simulink model "stormAD_Architecture_v1"  (R2024a)
settings: Solver=FixedStepDiscrete  StartTime=0.0  StopTime=10.0  RelTol=1e-3
model workspace (MAT data in the model file):
  bstInterface : Simulink.Bus (value not decoded)
undefined symbols (not defined in the file): orig, RepoFilePath, UI, VisualizeDataset
(part 2 of 3)

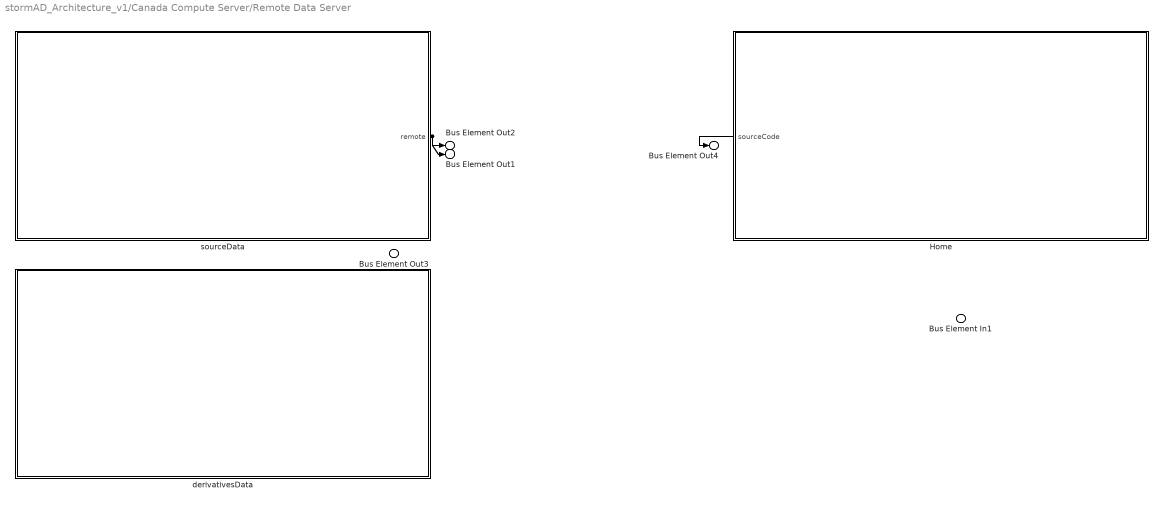
== system stormAD_Architecture_v1/Canada Compute Server/Remote Data Server ==
  Bus Element In1 : Inport  PortName=Derivatives
  " sourceData" : Subsystem
      settings: PortSchema="{\"entries\":[{\"content\":{\"headerSize\":26,\"margin\":15,\"minimumSpacing\":25,\"sides\":[{\"content\":{},\"type\":\"ConnectorPlacement.EquallySpacedRectSide\",\"uuid\":\"a3539b9a-22db-4da3-b271-35b287ced3a1\"},{\"content\":{\"connectorIds\":[\"Out1\"],\"side\":\"RIGHT\"},\"type\":\"ConnectorPlacement.EquallySpacedRectSide\",\"uuid\":\"72d9f298-5062-46d4-b3c5-f2fa85d7a7a6\"},{\"content\":{\"side\":\"TOP\"},\"type\":\"ConnectorPlacement.EquallySpacedRectSide\",\"uuid\":\"050469fd-3881-4b53-a813-94df038aa659\"}]},\"type\":\"ConnectorPlacement.EquallySpacedConnector\",\"uuid\":\"6db04dad-62f3-4987-a6a9-d236db4fe2a3\"}],\"packageUris\":[\"http://schema.mathworks.com/mf0/Connector/R2020b\"],\"version\":\"1.0\"}"
  Home : Subsystem
      settings: PortSchema="{\"entries\":[{\"content\":{\"headerSize\":26,\"margin\":15,\"minimumSpacing\":25,\"sides\":[{\"content\":{\"connectorIds\":[\"Out1\"]},\"type\":\"ConnectorPlacement.EquallySpacedRectSide\",\"uuid\":\"a3539b9a-22db-4da3-b271-35b287ced3a1\"},{\"content\":{\"side\":\"RIGHT\"},\"type\":\"ConnectorPlacement.EquallySpacedRectSide\",\"uuid\":\"72d9f298-5062-46d4-b3c5-f2fa85d7a7a6\"},{\"content\":{\"side\":\"TOP\"},\"type\":\"ConnectorPlacement.EquallySpacedRectSide\",\"uuid\":\"050469fd-3881-4b53-a813-94df038aa659\"}]},\"type\":\"ConnectorPlacement.EquallySpacedConnector\",\"uuid\":\"6db04dad-62f3-4987-a6a9-d236db4fe2a3\"}],\"packageUris\":[\"http://schema.mathworks.com/mf0/Connector/R2020b\"],\"version\":\"1.0\"}"
  derivativesData : Subsystem
      settings: PortSchema="{\"entries\":[{\"content\":{\"headerSize\":26,\"margin\":15,\"minimumSpacing\":25,\"sides\":[{\"content\":{},\"type\":\"ConnectorPlacement.EquallySpacedRectSide\",\"uuid\":\"a3539b9a-22db-4da3-b271-35b287ced3a1\"},{\"content\":{\"side\":\"RIGHT\"},\"type\":\"ConnectorPlacement.EquallySpacedRectSide\",\"uuid\":\"72d9f298-5062-46d4-b3c5-f2fa85d7a7a6\"},{\"content\":{\"side\":\"TOP\"},\"type\":\"ConnectorPlacement.EquallySpacedRectSide\",\"uuid\":\"050469fd-3881-4b53-a813-94df038aa659\"}]},\"type\":\"ConnectorPlacement.EquallySpacedConnector\",\"uuid\":\"6db04dad-62f3-4987-a6a9-d236db4fe2a3\"}],\"packageUris\":[\"http://schema.mathworks.com/mf0/Connector/R2020b\"],\"version\":\"1.0\"}"
  Bus Element Out4 : Outport  AllowServiceAccess=on  PortName=sourceCode  Element=github
  Bus Element Out3 : Outport  Port=2  AllowServiceAccess=on  PortName=SSHPort
  Bus Element Out1 : Outport  Port=3  AllowServiceAccess=on  PortName=remote.raw
  Bus Element Out2 : Outport  Port=4  AllowServiceAccess=on  PortName=remote.derivatives
  wires:
  " sourceData"/1(remote) -> Bus Element Out1/1, Bus Element Out2/1
  Home/1(sourceCode) -> Bus Element Out4/1

== system stormAD_Architecture_v1/Canada Compute Server/create Virtual Environment ==

== system stormAD_Architecture_v1/Canada Compute Server/gitClone Brainstorm ==
  Bus Element In1 : Inport  AllowServiceAccess=on  PortName=sourceCode

== system stormAD_Architecture_v1/Canada Compute Server/jobScheduler ==

== system stormAD_Architecture_v1/Canada Compute Server/loadPython ==

== system stormAD_Architecture_v1/Canada Compute Server/processingSoftware ==

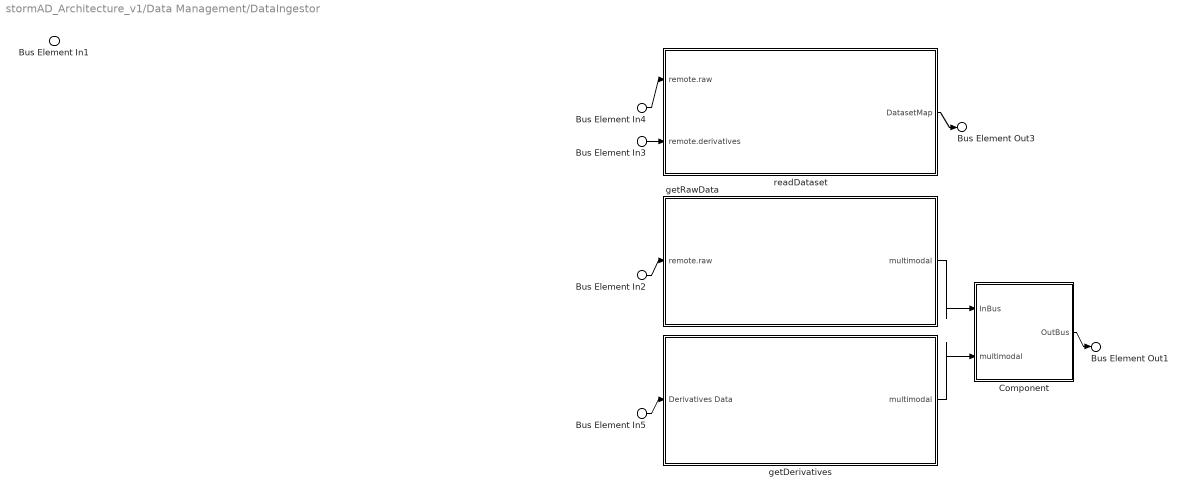
== system stormAD_Architecture_v1/Data Management/DataIngestor ==
  Bus Element In2 : Inport  AllowServiceAccess=on  PortName=remote.raw
  Bus Element In4 : Inport  AllowServiceAccess=on  PortName=remote.raw
  Bus Element In3 : Inport  Port=2  AllowServiceAccess=on  PortName=remote.derivatives
  Bus Element In5 : Inport  Port=2  AllowServiceAccess=on  PortName=remote.derivatives
  Bus Element In1 : Inport  Port=3  PortName=DataRequest
  Component : Subsystem
      settings: PortSchema="{\"entries\":[{\"content\":{\"headerSize\":26,\"margin\":15,\"minimumSpacing\":25,\"sides\":[{\"content\":{\"connectorIds\":[\"In1\",\"In2\"]},\"type\":\"ConnectorPlacement.EquallySpacedRectSide\",\"uuid\":\"a3539b9a-22db-4da3-b271-35b287ced3a1\"},{\"content\":{\"connectorIds\":[\"Out1\"],\"side\":\"RIGHT\"},\"type\":\"ConnectorPlacement.EquallySpacedRectSide\",\"uuid\":\"72d9f298-5062-46d4-b3c5-f2fa85d7a7a6\"},{\"content\":{\"side\":\"TOP\"},\"type\":\"ConnectorPlacement.EquallySpacedRectSide\",\"uuid\":\"050469fd-3881-4b53-a813-94df038aa659\"}]},\"type\":\"ConnectorPlacement.EquallySpacedConnector\",\"uuid\":\"6db04dad-62f3-4987-a6a9-d236db4fe2a3\"}],\"packageUris\":[\"http://schema.mathworks.com/mf0/Connector/R2020b\"],\"version\":\"1.0\"}"
  getDerivatives : Subsystem
      settings: PortSchema="{\"entries\":[{\"content\":{\"headerSize\":26,\"margin\":15,\"minimumSpacing\":25,\"sides\":[{\"content\":{\"connectorIds\":[\"In1\"]},\"type\":\"ConnectorPlacement.EquallySpacedRectSide\",\"uuid\":\"d99db108-8c8a-4010-81b2-f142fbf318f5\"},{\"content\":{\"connectorIds\":[\"Out1\"],\"side\":\"RIGHT\"},\"type\":\"ConnectorPlacement.EquallySpacedRectSide\",\"uuid\":\"9190d96c-22e3-4cc9-a507-8f094dc67743\"},{\"content\":{\"side\":\"TOP\"},\"type\":\"ConnectorPlacement.EquallySpacedRectSide\",\"uuid\":\"08b46875-eac1-4edb-b2eb-5598dd517a75\"}]},\"type\":\"ConnectorPlacement.EquallySpacedConnector\",\"uuid\":\"c8d2d02b-cf5a-431f-8876-22d36c8a9b33\"}],\"packageUris\":[\"http://schema.mathworks.com/mf0/Connector/R2020b\"],\"version\":\"1.0\"}"
  getRawData : Subsystem
      settings: PortSchema="{\"entries\":[{\"content\":{\"headerSize\":26,\"margin\":15,\"minimumSpacing\":25,\"sides\":[{\"content\":{\"connectorIds\":[\"In1\"]},\"type\":\"ConnectorPlacement.EquallySpacedRectSide\",\"uuid\":\"d99db108-8c8a-4010-81b2-f142fbf318f5\"},{\"content\":{\"connectorIds\":[\"Out1\"],\"side\":\"RIGHT\"},\"type\":\"ConnectorPlacement.EquallySpacedRectSide\",\"uuid\":\"9190d96c-22e3-4cc9-a507-8f094dc67743\"},{\"content\":{\"side\":\"TOP\"},\"type\":\"ConnectorPlacement.EquallySpacedRectSide\",\"uuid\":\"08b46875-eac1-4edb-b2eb-5598dd517a75\"}]},\"type\":\"ConnectorPlacement.EquallySpacedConnector\",\"uuid\":\"c8d2d02b-cf5a-431f-8876-22d36c8a9b33\"}],\"packageUris\":[\"http://schema.mathworks.com/mf0/Connector/R2020b\"],\"version\":\"1.0\"}"
  readDataset : Subsystem
      settings: PortSchema="{\"entries\":[{\"content\":{\"headerSize\":26,\"margin\":15,\"minimumSpacing\":25,\"sides\":[{\"content\":{\"connectorIds\":[\"In1\",\"In2\"]},\"type\":\"ConnectorPlacement.EquallySpacedRectSide\",\"uuid\":\"d99db108-8c8a-4010-81b2-f142fbf318f5\"},{\"content\":{\"connectorIds\":[\"Out1\"],\"side\":\"RIGHT\"},\"type\":\"ConnectorPlacement.EquallySpacedRectSide\",\"uuid\":\"9190d96c-22e3-4cc9-a507-8f094dc67743\"},{\"content\":{\"side\":\"TOP\"},\"type\":\"ConnectorPlacement.EquallySpacedRectSide\",\"uuid\":\"08b46875-eac1-4edb-b2eb-5598dd517a75\"}]},\"type\":\"ConnectorPlacement.EquallySpacedConnector\",\"uuid\":\"c8d2d02b-cf5a-431f-8876-22d36c8a9b33\"}],\"packageUris\":[\"http://schema.mathworks.com/mf0/Connector/R2020b\"],\"version\":\"1.0\"}"
  Bus Element Out1 : Outport  PortName=remote
  Bus Element Out3 : Outport  Port=2  PortName=DatasetMap
  wires:
  readDataset/1(DatasetMap) -> Bus Element Out3/1
  Bus Element In2/1 -> getRawData/1(remote.raw)
  Bus Element In4/1 -> readDataset/1(remote.raw)
  Bus Element In3/1 -> readDataset/2(remote.derivatives)
  Bus Element In5/1 -> getDerivatives/1(Derivatives Data)
  getDerivatives/1(multimodal) -> Component/2(multimodal)
  getRawData/1(multimodal) -> Component/1(InBus)
  Component/1(OutBus) -> Bus Element Out1/1

== system stormAD_Architecture_v1/Data Management/Database Server ==
  Bus Element In2 : Inport  PortName=DerivativesMetadata
  Bus Element In3 : Inport  Port=2  PortName=Local Derivatives Metadata
  Bus Element In1 : Inport  Port=3  PortName=Dataset Metadata
  Bus Element Out1 : Outport  AllowServiceAccess=on  PortName=Metadata

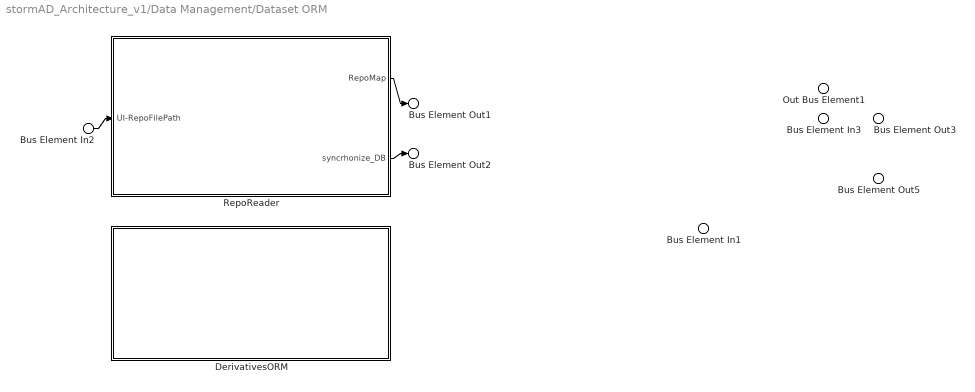
== system stormAD_Architecture_v1/Data Management/Dataset ORM ==
  Bus Element In3 : Inport  PortName=DatasetMap
  Bus Element In2 : Inport  Port=2  PortName=UI-RepoFilePath
  Bus Element In1 : Inport  Port=3  AllowServiceAccess=on  PortName=Metadata
  DerivativesORM : Subsystem
      settings: PortSchema="{\"entries\":[{\"content\":{\"headerSize\":26,\"margin\":15,\"minimumSpacing\":25,\"sides\":[{\"content\":{},\"type\":\"ConnectorPlacement.EquallySpacedRectSide\",\"uuid\":\"d99db108-8c8a-4010-81b2-f142fbf318f5\"},{\"content\":{\"side\":\"RIGHT\"},\"type\":\"ConnectorPlacement.EquallySpacedRectSide\",\"uuid\":\"9190d96c-22e3-4cc9-a507-8f094dc67743\"},{\"content\":{\"side\":\"TOP\"},\"type\":\"ConnectorPlacement.EquallySpacedRectSide\",\"uuid\":\"08b46875-eac1-4edb-b2eb-5598dd517a75\"}]},\"type\":\"ConnectorPlacement.EquallySpacedConnector\",\"uuid\":\"c8d2d02b-cf5a-431f-8876-22d36c8a9b33\"}],\"packageUris\":[\"http://schema.mathworks.com/mf0/Connector/R2020b\"],\"version\":\"1.0\"}"
  RepoReader : Subsystem
      settings: PortSchema="{\"entries\":[{\"content\":{\"headerSize\":26,\"margin\":15,\"minimumSpacing\":25,\"sides\":[{\"content\":{\"connectorIds\":[\"In1\"]},\"type\":\"ConnectorPlacement.EquallySpacedRectSide\",\"uuid\":\"d99db108-8c8a-4010-81b2-f142fbf318f5\"},{\"content\":{\"connectorIds\":[\"Out1\",\"Out2\"],\"side\":\"RIGHT\"},\"type\":\"ConnectorPlacement.EquallySpacedRectSide\",\"uuid\":\"9190d96c-22e3-4cc9-a507-8f094dc67743\"},{\"content\":{\"side\":\"TOP\"},\"type\":\"ConnectorPlacement.EquallySpacedRectSide\",\"uuid\":\"08b46875-eac1-4edb-b2eb-5598dd517a75\"}]},\"type\":\"ConnectorPlacement.EquallySpacedConnector\",\"uuid\":\"c8d2d02b-cf5a-431f-8876-22d36c8a9b33\"}],\"packageUris\":[\"http://schema.mathworks.com/mf0/Connector/R2020b\"],\"version\":\"1.0\"}"
  Bus Element Out5 : Outport  PortName=DerivativesMetadata
  Bus Element Out2 : Outport  Port=2  PortName=syncrhonize_DB
  Bus Element Out3 : Outport  Port=3  PortName=DataRequest
  Bus Element Out1 : Outport  Port=4  PortName=RepoMap
  Out Bus Element1 : Outport  Port=5  PortName=UI-VisualizeDataset
  wires:
  Bus Element In2/1 -> RepoReader/1(UI-RepoFilePath)
  RepoReader/1(RepoMap) -> Bus Element Out1/1
  RepoReader/2(syncrhonize_DB) -> Bus Element Out2/1

== system stormAD_Architecture_v1/Local Data Server/UserDir ==
  Bus Element Out1 : Outport  AllowServiceAccess=on  PortName=userConfigRemote

== system stormAD_Architecture_v1/Local Data Server/brainstorm3 ==

== system stormAD_Architecture_v1/Local Data Server/brainstorm_db ==
  Bus Element In1 : Inport  AllowServiceAccess=on  PortName=Derivatives

== system stormAD_Architecture_v1/Local Data Server/remoteConfig ==
  Bus Element Out1 : Outport  AllowServiceAccess=on  PortName=userConfigRemote

== system stormAD_Architecture_v1/Local Data Server/sourceData ==
  Bus Element In2 : Inport  AllowServiceAccess=on  PortName=StormDerivatives
  Bus Element In1 : Inport  Port=2  PortName=remote
  Out Bus Element1 : Outport  PortName=local

== system stormAD_Architecture_v1/Remote Data Connect/LORIS Data Ingestor ==

== system stormAD_Architecture_v1/Remote Data Connect/Linux ==
  Bus Element In1 : Inport  AllowServiceAccess=on  PortName=Client

== system stormAD_Architecture_v1/Remote Data Connect/Windows ==
  Bus Element In1 : Inport  AllowServiceAccess=on  PortName=Client

== system stormAD_Architecture_v1/Remote Data Connect/gitClone Brainstorm ==
  Bus Element In1 : Inport  AllowServiceAccess=on  PortName=sourceCode

== system stormAD_Architecture_v1/StormAD Core/Anatomy ==
  Bus Element In1 : Inport  PortName=anat
  Bus Element Out1 : Outport  PortName=anat4pet
  Bus Element Out2 : Outport  Port=2  PortName=anat4meg
  Bus Element Out3 : Outport  Port=3  PortName=anatMetadata
  Bus Element Out4 : Outport  Port=4  PortName=anatDerivs

== system stormAD_Architecture_v1/StormAD Core/MEG ==
  Bus Element In2 : Inport  PortName=anat4meg
  Bus Element In1 : Inport  Port=2  PortName=meg
  featureExtractionModule : Subsystem
      settings: PortSchema="{\"entries\":[{\"content\":{\"headerSize\":26,\"margin\":15,\"minimumSpacing\":25,\"sides\":[{\"content\":{},\"type\":\"ConnectorPlacement.EquallySpacedRectSide\",\"uuid\":\"a3539b9a-22db-4da3-b271-35b287ced3a1\"},{\"content\":{\"side\":\"RIGHT\"},\"type\":\"ConnectorPlacement.EquallySpacedRectSide\",\"uuid\":\"72d9f298-5062-46d4-b3c5-f2fa85d7a7a6\"},{\"content\":{\"side\":\"TOP\"},\"type\":\"ConnectorPlacement.EquallySpacedRectSide\",\"uuid\":\"050469fd-3881-4b53-a813-94df038aa659\"}]},\"type\":\"ConnectorPlacement.EquallySpacedConnector\",\"uuid\":\"6db04dad-62f3-4987-a6a9-d236db4fe2a3\"}],\"packageUris\":[\"http://schema.mathworks.com/mf0/Connector/R2020b\"],\"version\":\"1.0\"}"
  Bus Element Out1 : Outport  PortName=megMetadata
  Bus Element Out2 : Outport  Port=2  PortName=megSurf
  Bus Element Out3 : Outport  Port=3  PortName=megDerivs

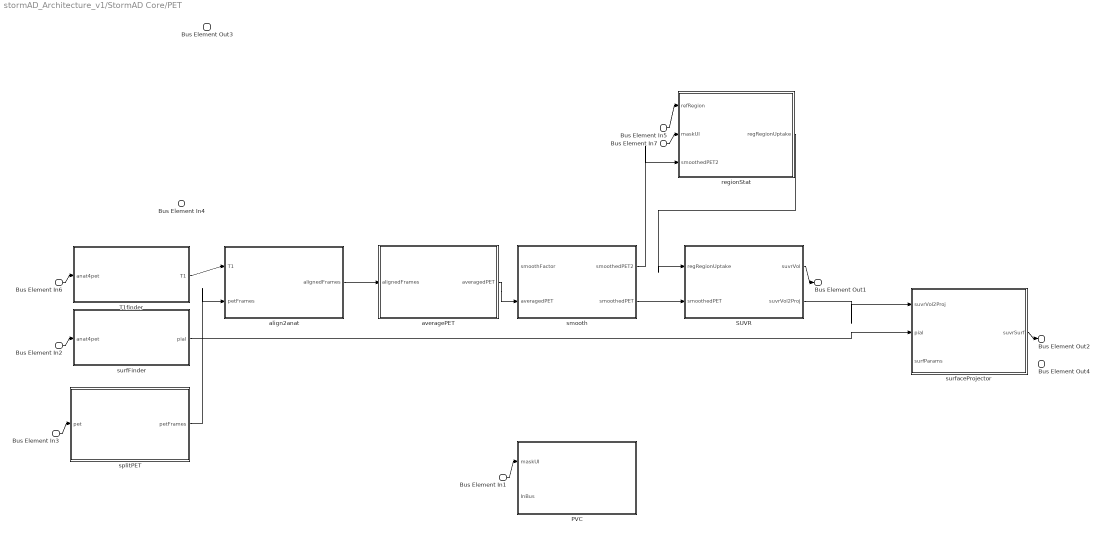
== system stormAD_Architecture_v1/StormAD Core/PET ==
  Bus Element In7 : Inport  PortName=maskUI
  Bus Element In1 : Inport  PortName=maskUI
  Bus Element In5 : Inport  Port=2  PortName=anat4pet
  Bus Element In6 : Inport  Port=2  PortName=anat4pet
  Bus Element In2 : Inport  Port=2  PortName=anat4pet
  Bus Element In4 : Inport  Port=2  PortName=anat4pet  Element=signal1
  Bus Element In3 : Inport  Port=3  PortName=pet
  PVC : Subsystem
      settings: PortSchema="{\"entries\":[{\"content\":{\"headerSize\":26,\"margin\":15,\"minimumSpacing\":25,\"sides\":[{\"content\":{\"connectorIds\":[\"In1\",\"In2\"]},\"type\":\"ConnectorPlacement.EquallySpacedRectSide\",\"uuid\":\"a3539b9a-22db-4da3-b271-35b287ced3a1\"},{\"content\":{\"side\":\"RIGHT\"},\"type\":\"ConnectorPlacement.EquallySpacedRectSide\",\"uuid\":\"72d9f298-5062-46d4-b3c5-f2fa85d7a7a6\"},{\"content\":{\"side\":\"TOP\"},\"type\":\"ConnectorPlacement.EquallySpacedRectSide\",\"uuid\":\"050469fd-3881-4b53-a813-94df038aa659\"}]},\"type\":\"ConnectorPlacement.EquallySpacedConnector\",\"uuid\":\"6db04dad-62f3-4987-a6a9-d236db4fe2a3\"}],\"packageUris\":[\"http://schema.mathworks.com/mf0/Connector/R2020b\"],\"version\":\"1.0\"}"
  SUVR : Subsystem
      settings: PortSchema="{\"entries\":[{\"content\":{\"headerSize\":26,\"margin\":15,\"minimumSpacing\":25,\"sides\":[{\"content\":{\"connectorIds\":[\"In1\",\"In2\"]},\"type\":\"ConnectorPlacement.EquallySpacedRectSide\",\"uuid\":\"a3539b9a-22db-4da3-b271-35b287ced3a1\"},{\"content\":{\"connectorIds\":[\"Out1\",\"Out2\"],\"side\":\"RIGHT\"},\"type\":\"ConnectorPlacement.EquallySpacedRectSide\",\"uuid\":\"72d9f298-5062-46d4-b3c5-f2fa85d7a7a6\"},{\"content\":{\"side\":\"TOP\"},\"type\":\"ConnectorPlacement.EquallySpacedRectSide\",\"uuid\":\"050469fd-3881-4b53-a813-94df038aa659\"}]},\"type\":\"ConnectorPlacement.EquallySpacedConnector\",\"uuid\":\"6db04dad-62f3-4987-a6a9-d236db4fe2a3\"}],\"packageUris\":[\"http://schema.mathworks.com/mf0/Connector/R2020b\"],\"version\":\"1.0\"}"
  T1finder : Subsystem
      settings: PortSchema="{\"entries\":[{\"content\":{\"headerSize\":26,\"margin\":15,\"minimumSpacing\":25,\"sides\":[{\"content\":{\"connectorIds\":[\"In1\"]},\"type\":\"ConnectorPlacement.EquallySpacedRectSide\",\"uuid\":\"a3539b9a-22db-4da3-b271-35b287ced3a1\"},{\"content\":{\"connectorIds\":[\"Out1\"],\"side\":\"RIGHT\"},\"type\":\"ConnectorPlacement.EquallySpacedRectSide\",\"uuid\":\"72d9f298-5062-46d4-b3c5-f2fa85d7a7a6\"},{\"content\":{\"side\":\"TOP\"},\"type\":\"ConnectorPlacement.EquallySpacedRectSide\",\"uuid\":\"050469fd-3881-4b53-a813-94df038aa659\"},{\"content\":{\"side\":\"BOTTOM\"},\"type\":\"ConnectorPlacement.EquallySpacedRectSide\",\"uuid\":\"a1469e70-16e5-4ce1-b6fd-4b50fed9e5f8\"}]},\"type\":\"ConnectorPlacement.EquallySpacedConnector\",\"uuid\":\"6db04dad-62f3-4987-a6a9-d236db4fe2a3\"}],\"packageUris\":[\"http://schema.mathworks.com/mf0/Connector/R2020b\"],\"version\":\"1.0\"}"
  align2anat : Subsystem
      settings: PortSchema="{\"entries\":[{\"content\":{\"headerSize\":26,\"margin\":15,\"minimumSpacing\":25,\"sides\":[{\"content\":{\"connectorIds\":[\"In1\",\"In2\"]},\"type\":\"ConnectorPlacement.EquallySpacedRectSide\",\"uuid\":\"a3539b9a-22db-4da3-b271-35b287ced3a1\"},{\"content\":{\"connectorIds\":[\"Out1\"],\"side\":\"RIGHT\"},\"type\":\"ConnectorPlacement.EquallySpacedRectSide\",\"uuid\":\"72d9f298-5062-46d4-b3c5-f2fa85d7a7a6\"},{\"content\":{\"side\":\"TOP\"},\"type\":\"ConnectorPlacement.EquallySpacedRectSide\",\"uuid\":\"050469fd-3881-4b53-a813-94df038aa659\"}]},\"type\":\"ConnectorPlacement.EquallySpacedConnector\",\"uuid\":\"6db04dad-62f3-4987-a6a9-d236db4fe2a3\"}],\"packageUris\":[\"http://schema.mathworks.com/mf0/Connector/R2020b\"],\"version\":\"1.0\"}"
  averagePET : Subsystem
      settings: PortSchema="{\"entries\":[{\"content\":{\"headerSize\":26,\"margin\":15,\"minimumSpacing\":25,\"sides\":[{\"content\":{\"connectorIds\":[\"In1\"]},\"type\":\"ConnectorPlacement.EquallySpacedRectSide\",\"uuid\":\"a3539b9a-22db-4da3-b271-35b287ced3a1\"},{\"content\":{\"connectorIds\":[\"Out1\"],\"side\":\"RIGHT\"},\"type\":\"ConnectorPlacement.EquallySpacedRectSide\",\"uuid\":\"72d9f298-5062-46d4-b3c5-f2fa85d7a7a6\"},{\"content\":{\"side\":\"TOP\"},\"type\":\"ConnectorPlacement.EquallySpacedRectSide\",\"uuid\":\"050469fd-3881-4b53-a813-94df038aa659\"}]},\"type\":\"ConnectorPlacement.EquallySpacedConnector\",\"uuid\":\"6db04dad-62f3-4987-a6a9-d236db4fe2a3\"}],\"packageUris\":[\"http://schema.mathworks.com/mf0/Connector/R2020b\"],\"version\":\"1.0\"}"
  regionStat : Subsystem
      settings: PortSchema="{\"entries\":[{\"content\":{\"headerSize\":26,\"margin\":15,\"minimumSpacing\":25,\"sides\":[{\"content\":{\"connectorIds\":[\"In1\",\"In2\",\"In3\"]},\"type\":\"ConnectorPlacement.EquallySpacedRectSide\",\"uuid\":\"a3539b9a-22db-4da3-b271-35b287ced3a1\"},{\"content\":{\"connectorIds\":[\"Out1\"],\"side\":\"RIGHT\"},\"type\":\"ConnectorPlacement.EquallySpacedRectSide\",\"uuid\":\"72d9f298-5062-46d4-b3c5-f2fa85d7a7a6\"},{\"content\":{\"side\":\"TOP\"},\"type\":\"ConnectorPlacement.EquallySpacedRectSide\",\"uuid\":\"050469fd-3881-4b53-a813-94df038aa659\"}]},\"type\":\"ConnectorPlacement.EquallySpacedConnector\",\"uuid\":\"6db04dad-62f3-4987-a6a9-d236db4fe2a3\"}],\"packageUris\":[\"http://schema.mathworks.com/mf0/Connector/R2020b\"],\"version\":\"1.0\"}"
  smooth : Subsystem
      settings: PortSchema="{\"entries\":[{\"content\":{\"headerSize\":26,\"margin\":15,\"minimumSpacing\":25,\"sides\":[{\"content\":{\"connectorIds\":[\"In1\",\"In2\"]},\"type\":\"ConnectorPlacement.EquallySpacedRectSide\",\"uuid\":\"a3539b9a-22db-4da3-b271-35b287ced3a1\"},{\"content\":{\"connectorIds\":[\"Out1\",\"Out2\"],\"side\":\"RIGHT\"},\"type\":\"ConnectorPlacement.EquallySpacedRectSide\",\"uuid\":\"72d9f298-5062-46d4-b3c5-f2fa85d7a7a6\"},{\"content\":{\"side\":\"TOP\"},\"type\":\"ConnectorPlacement.EquallySpacedRectSide\",\"uuid\":\"050469fd-3881-4b53-a813-94df038aa659\"}]},\"type\":\"ConnectorPlacement.EquallySpacedConnector\",\"uuid\":\"6db04dad-62f3-4987-a6a9-d236db4fe2a3\"}],\"packageUris\":[\"http://schema.mathworks.com/mf0/Connector/R2020b\"],\"version\":\"1.0\"}"
  splitPET : Subsystem
      settings: PortSchema="{\"entries\":[{\"content\":{\"headerSize\":26,\"margin\":15,\"minimumSpacing\":25,\"sides\":[{\"content\":{\"connectorIds\":[\"In1\"]},\"type\":\"ConnectorPlacement.EquallySpacedRectSide\",\"uuid\":\"a3539b9a-22db-4da3-b271-35b287ced3a1\"},{\"content\":{\"connectorIds\":[\"Out1\"],\"side\":\"RIGHT\"},\"type\":\"ConnectorPlacement.EquallySpacedRectSide\",\"uuid\":\"72d9f298-5062-46d4-b3c5-f2fa85d7a7a6\"},{\"content\":{\"side\":\"TOP\"},\"type\":\"ConnectorPlacement.EquallySpacedRectSide\",\"uuid\":\"050469fd-3881-4b53-a813-94df038aa659\"}]},\"type\":\"ConnectorPlacement.EquallySpacedConnector\",\"uuid\":\"6db04dad-62f3-4987-a6a9-d236db4fe2a3\"}],\"packageUris\":[\"http://schema.mathworks.com/mf0/Connector/R2020b\"],\"version\":\"1.0\"}"
  surfFinder : Subsystem
      settings: PortSchema="{\"entries\":[{\"content\":{\"headerSize\":26,\"margin\":15,\"minimumSpacing\":25,\"sides\":[{\"content\":{\"connectorIds\":[\"In1\"]},\"type\":\"ConnectorPlacement.EquallySpacedRectSide\",\"uuid\":\"a3539b9a-22db-4da3-b271-35b287ced3a1\"},{\"content\":{\"connectorIds\":[\"Out1\"],\"side\":\"RIGHT\"},\"type\":\"ConnectorPlacement.EquallySpacedRectSide\",\"uuid\":\"72d9f298-5062-46d4-b3c5-f2fa85d7a7a6\"},{\"content\":{\"side\":\"TOP\"},\"type\":\"ConnectorPlacement.EquallySpacedRectSide\",\"uuid\":\"050469fd-3881-4b53-a813-94df038aa659\"}]},\"type\":\"ConnectorPlacement.EquallySpacedConnector\",\"uuid\":\"6db04dad-62f3-4987-a6a9-d236db4fe2a3\"}],\"packageUris\":[\"http://schema.mathworks.com/mf0/Connector/R2020b\"],\"version\":\"1.0\"}"
  surfaceProjector : Subsystem
      settings: PortSchema="{\"entries\":[{\"content\":{\"headerSize\":26,\"margin\":15,\"minimumSpacing\":25,\"sides\":[{\"content\":{\"connectorIds\":[\"In1\",\"In3\",\"In2\"]},\"type\":\"ConnectorPlacement.EquallySpacedRectSide\",\"uuid\":\"a3539b9a-22db-4da3-b271-35b287ced3a1\"},{\"content\":{\"connectorIds\":[\"Out1\"],\"side\":\"RIGHT\"},\"type\":\"ConnectorPlacement.EquallySpacedRectSide\",\"uuid\":\"72d9f298-5062-46d4-b3c5-f2fa85d7a7a6\"},{\"content\":{\"side\":\"TOP\"},\"type\":\"ConnectorPlacement.EquallySpacedRectSide\",\"uuid\":\"050469fd-3881-4b53-a813-94df038aa659\"},{\"content\":{\"side\":\"BOTTOM\"},\"type\":\"ConnectorPlacement.EquallySpacedRectSide\",\"uuid\":\"ca80c562-ab11-42f8-9713-788a61e6aac3\"}]},\"type\":\"ConnectorPlacement.EquallySpacedConnector\",\"uuid\":\"6db04dad-62f3-4987-a6a9-d236db4fe2a3\"}],\"packageUris\":[\"http://schema.mathworks.com/mf0/Connector/R2020b\"],\"version\":\"1.0\"}"
  Bus Element Out3 : Outport  PortName=petMedata
  Bus Element Out1 : Outport  Port=2  PortName=suvrVol
  Bus Element Out2 : Outport  Port=3  PortName=suvrSurf
  Bus Element Out4 : Outport  Port=4  PortName=petDerivs
  wires:
  Bus Element In3/1 -> splitPET/1(pet)
  splitPET/1(petFrames) -> align2anat/2(petFrames)
  align2anat/1(alignedFrames) -> averagePET/1(alignedFrames)
  averagePET/1(averagedPET) -> smooth/2(averagedPET)
  smooth/2(smoothedPET) -> SUVR/2(smoothedPET)
  Bus Element In5/1 -> regionStat/1(refRegion)
  regionStat/1(regRegionUptake) -> SUVR/1(regRegionUptake)
  Bus Element In6/1 -> T1finder/1(anat4pet)
  T1finder/1(T1) -> align2anat/1(T1)
  smooth/1(smoothedPET2) -> regionStat/3(smoothedPET2)
  Bus Element In7/1 -> regionStat/2(maskUI)
  Bus Element In1/1 -> PVC/1(maskUI)
  Bus Element In2/1 -> surfFinder/1(anat4pet)
  surfFinder/1(pial) -> surfaceProjector/3(pial)
  SUVR/1(suvrVol) -> Bus Element Out1/1
  SUVR/2(suvrVol2Proj) -> surfaceProjector/1(suvrVol2Proj)
  surfaceProjector/1(suvrSurf) -> Bus Element Out2/1

== system stormAD_Architecture_v1/StormAD Core/UserConfig ==
  Bus Element In1 : Inport  PortName=bstConfig

== system stormAD_Architecture_v1/StormAD Core/dataAllocator ==
  Bus Element In1 : Inport  AllowServiceAccess=on  PortName=Data
  Bus Element Out1 : Outport  PortName=anat
  Bus Element Out2 : Outport  Port=2  PortName=pet
  Bus Element Out3 : Outport  Port=3  PortName=meg

== system stormAD_Architecture_v1/StormAD Core/derivsRouter ==
  Bus Element In1 : Inport  PortName=petDerivs
  Bus Element In3 : Inport  Port=2  PortName=anatDerivs
  Bus Element In2 : Inport  Port=3  PortName=megDerivs
  Bus Element Out1 : Outport  AllowServiceAccess=on  PortName=BIDSDatasets

== system stormAD_Architecture_v1/StormAD Core/derivsTracker ==
  Bus Element In1 : Inport  PortName=petMetadata
  Bus Element In2 : Inport  Port=2  PortName=megMetadata
  Bus Element In3 : Inport  Port=3  PortName=anatMetadata
  Bus Element Out1 : Outport  AllowServiceAccess=on  PortName=Derivatives Metadata

== system stormAD_Architecture_v1/StormAD Core/importBIDSDataset ==
  Bus Element In1 : Inport  AllowServiceAccess=on  PortName=local.raw
  Bus Element Out1 : Outport  AllowServiceAccess=on  PortName=Derivatives

== system stormAD_Architecture_v1/StormAD Interface/Local Cache1 ==
  Bus Element In1 : Inport  PortName=convertedData
  Bus Element In2 : Inport  Port=2  PortName=freesurfer_derivatives
  Bus Element Out2 : Outport  PortName=Local Derivatives Metadata
  Bus Element Out3 : Outport  Port=2  PortName=orig
  Bus Element Out1 : Outport  Port=3  PortName=Local Derivatives

== system stormAD_Architecture_v1/StormAD Interface/availableDatasetsUI ==
  Bus Element In1 : Inport  PortName=datasetMap
  Bus Element Out1 : Outport  PortName=UI

== system stormAD_Architecture_v1/StormAD Interface/ingestData ==
  Bus Element In1 : Inport  PortName=UI
  Bus Element In2 : Inport  Port=2  PortName=Data
  Bus Element Out1 : Outport  PortName=convertedData

== system stormAD_Architecture_v1/StormAD Remote/Local WSL Store ==
  Bus Element In2 : Inport  PortName=win2wsl
  bash Scripts : Subsystem
      settings: PortSchema="{\"entries\":[{\"content\":{\"headerSize\":26,\"margin\":15,\"minimumSpacing\":25,\"sides\":[{\"content\":{},\"type\":\"ConnectorPlacement.EquallySpacedRectSide\",\"uuid\":\"97c1e145-3d4b-49de-9739-71f2af5be190\"},{\"content\":{\"side\":\"RIGHT\"},\"type\":\"ConnectorPlacement.EquallySpacedRectSide\",\"uuid\":\"5a937baa-e46f-4764-8b00-75a1eb9e59b0\"},{\"content\":{\"side\":\"TOP\"},\"type\":\"ConnectorPlacement.EquallySpacedRectSide\",\"uuid\":\"83b91a39-9e34-441d-bccf-4f6b71aa9c87\"}]},\"type\":\"ConnectorPlacement.EquallySpacedConnector\",\"uuid\":\"3f7bec2f-99ca-4d64-b419-ed6b2efa51c2\"}],\"packageUris\":[\"http://schema.mathworks.com/mf0/Connector/R2020b\"],\"version\":\"1.0\"}"
  slurm Jobs : Subsystem
      settings: PortSchema="{\"entries\":[{\"content\":{\"headerSize\":26,\"margin\":15,\"minimumSpacing\":25,\"sides\":[{\"content\":{},\"type\":\"ConnectorPlacement.EquallySpacedRectSide\",\"uuid\":\"97c1e145-3d4b-49de-9739-71f2af5be190\"},{\"content\":{\"side\":\"RIGHT\"},\"type\":\"ConnectorPlacement.EquallySpacedRectSide\",\"uuid\":\"5a937baa-e46f-4764-8b00-75a1eb9e59b0\"},{\"content\":{\"side\":\"TOP\"},\"type\":\"ConnectorPlacement.EquallySpacedRectSide\",\"uuid\":\"83b91a39-9e34-441d-bccf-4f6b71aa9c87\"}]},\"type\":\"ConnectorPlacement.EquallySpacedConnector\",\"uuid\":\"3f7bec2f-99ca-4d64-b419-ed6b2efa51c2\"}],\"packageUris\":[\"http://schema.mathworks.com/mf0/Connector/R2020b\"],\"version\":\"1.0\"}"
  sshConnect : Subsystem
      settings: PortSchema="{\"entries\":[{\"content\":{\"headerSize\":26,\"margin\":15,\"minimumSpacing\":25,\"sides\":[{\"content\":{},\"type\":\"ConnectorPlacement.EquallySpacedRectSide\",\"uuid\":\"97c1e145-3d4b-49de-9739-71f2af5be190\"},{\"content\":{\"side\":\"RIGHT\"},\"type\":\"ConnectorPlacement.EquallySpacedRectSide\",\"uuid\":\"5a937baa-e46f-4764-8b00-75a1eb9e59b0\"},{\"content\":{\"side\":\"TOP\"},\"type\":\"ConnectorPlacement.EquallySpacedRectSide\",\"uuid\":\"83b91a39-9e34-441d-bccf-4f6b71aa9c87\"}]},\"type\":\"ConnectorPlacement.EquallySpacedConnector\",\"uuid\":\"3f7bec2f-99ca-4d64-b419-ed6b2efa51c2\"}],\"packageUris\":[\"http://schema.mathworks.com/mf0/Connector/R2020b\"],\"version\":\"1.0\"}"
  Bus Element Out2 : Outport  AllowServiceAccess=on  PortName=rsync
  Bus Element Out1 : Outport  Port=2  PortName=wsl2win

== system stormAD_Architecture_v1/StormAD Remote/Loris ==

== system stormAD_Architecture_v1/StormAD Remote/Remote Execution Module ==
  Bus Element In1 : Inport  AllowServiceAccess=on  PortName=SSHPort
  In Bus Element1 : Inport  Port=2  PortName=rsync

== system stormAD_Architecture_v1/StormAD Remote/SSH Connection Module ==
  Bus Element In2 : Inport  AllowServiceAccess=on  PortName=rsync
  Bus Element In1 : Inport  Port=2  AllowServiceAccess=on  PortName=SSHPort

== system stormAD_Architecture_v1/StormAD Remote/StormRemote GUI ==

== system stormAD_Architecture_v1/StormAD Remote/WSL Inteface Module ==
  Bus Element In2 : Inport  PortName=wsl2win
  Bus Element In1 : Inport  Port=2  AllowServiceAccess=on  PortName=remote.config
  Bus Element Out1 : Outport  PortName=win2wsl

== system stormAD_Architecture_v1/StormAD Remote/importBIDSDataset ==
  Bus Element In1 : Inport  AllowServiceAccess=on  PortName=local.raw
  Bus Element Out1 : Outport  AllowServiceAccess=on  PortName=Derivatives

== system stormAD_Architecture_v1/Canada Compute Server/Freesurfer Processing Server/PETSurfer ==
  Bus Element Out1 : Outport  PortName=pet

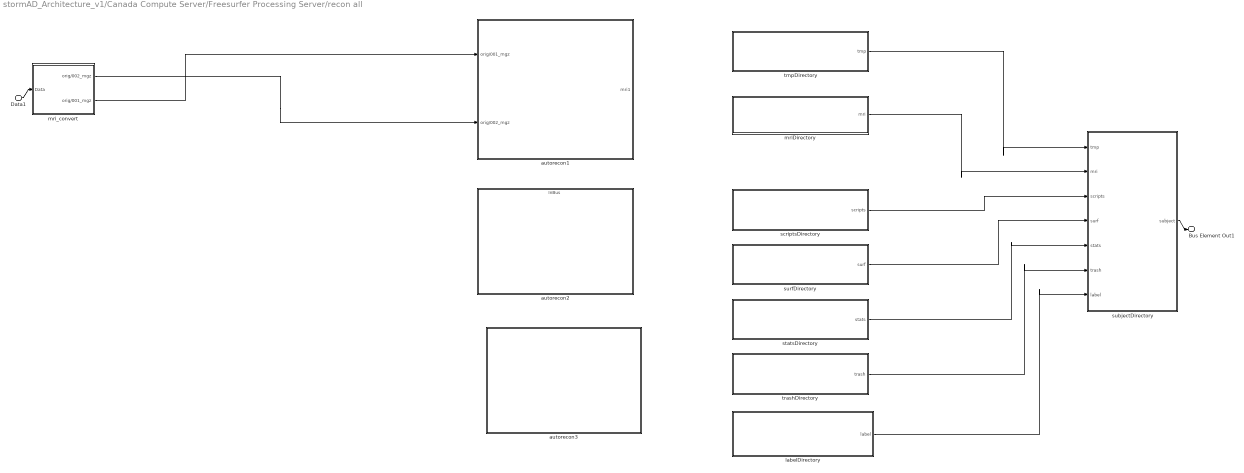
== system stormAD_Architecture_v1/Canada Compute Server/Freesurfer Processing Server/recon all ==
  Data1 : Inport  AllowServiceAccess=on  PortName=Data
  autorecon1 : Subsystem
      settings: PortSchema="{\"entries\":[{\"content\":{\"headerSize\":26,\"margin\":15,\"minimumSpacing\":25,\"sides\":[{\"content\":{\"connectorIds\":[\"In1\",\"In2\"]},\"type\":\"ConnectorPlacement.EquallySpacedRectSide\",\"uuid\":\"1ec5f43e-86ec-4420-9dd8-c30b843d5131\"},{\"content\":{\"connectorIds\":[\"Out1\"],\"side\":\"RIGHT\"},\"type\":\"ConnectorPlacement.EquallySpacedRectSide\",\"uuid\":\"372e8174-47dc-4989-909e-f78b7a521fdc\"},{\"content\":{\"side\":\"TOP\"},\"type\":\"ConnectorPlacement.EquallySpacedRectSide\",\"uuid\":\"cc67dfee-4023-44ab-9dd9-de9f078f7d77\"}]},\"type\":\"ConnectorPlacement.EquallySpacedConnector\",\"uuid\":\"fe3e41a6-8f67-44d2-abc6-74b481cf0464\"}],\"packageUris\":[\"http://schema.mathworks.com/mf0/Connector/R2020b\"],\"version\":\"1.0\"}"
  autorecon2 : Subsystem
      settings: PortSchema="{\"entries\":[{\"content\":{\"headerSize\":26,\"margin\":15,\"minimumSpacing\":25,\"sides\":[{\"content\":{},\"type\":\"ConnectorPlacement.EquallySpacedRectSide\",\"uuid\":\"d99db108-8c8a-4010-81b2-f142fbf318f5\"},{\"content\":{\"side\":\"RIGHT\"},\"type\":\"ConnectorPlacement.EquallySpacedRectSide\",\"uuid\":\"9190d96c-22e3-4cc9-a507-8f094dc67743\"},{\"content\":{\"connectorIds\":[\"In1\"],\"side\":\"TOP\"},\"type\":\"ConnectorPlacement.EquallySpacedRectSide\",\"uuid\":\"08b46875-eac1-4edb-b2eb-5598dd517a75\"}]},\"type\":\"ConnectorPlacement.EquallySpacedConnector\",\"uuid\":\"c8d2d02b-cf5a-431f-8876-22d36c8a9b33\"}],\"packageUris\":[\"http://schema.mathworks.com/mf0/Connector/R2020b\"],\"version\":\"1.0\"}"
  autorecon3 : Subsystem
      settings: PortSchema="{\"entries\":[{\"content\":{\"headerSize\":26,\"margin\":15,\"minimumSpacing\":25,\"sides\":[{\"content\":{},\"type\":\"ConnectorPlacement.EquallySpacedRectSide\",\"uuid\":\"d99db108-8c8a-4010-81b2-f142fbf318f5\"},{\"content\":{\"side\":\"RIGHT\"},\"type\":\"ConnectorPlacement.EquallySpacedRectSide\",\"uuid\":\"9190d96c-22e3-4cc9-a507-8f094dc67743\"},{\"content\":{\"side\":\"TOP\"},\"type\":\"ConnectorPlacement.EquallySpacedRectSide\",\"uuid\":\"08b46875-eac1-4edb-b2eb-5598dd517a75\"}]},\"type\":\"ConnectorPlacement.EquallySpacedConnector\",\"uuid\":\"c8d2d02b-cf5a-431f-8876-22d36c8a9b33\"}],\"packageUris\":[\"http://schema.mathworks.com/mf0/Connector/R2020b\"],\"version\":\"1.0\"}"
  labelDirectory : Subsystem
      settings: PortSchema="{\"entries\":[{\"content\":{\"headerSize\":26,\"margin\":15,\"minimumSpacing\":25,\"sides\":[{\"content\":{},\"type\":\"ConnectorPlacement.EquallySpacedRectSide\",\"uuid\":\"d99db108-8c8a-4010-81b2-f142fbf318f5\"},{\"content\":{\"connectorIds\":[\"Out1\"],\"side\":\"RIGHT\"},\"type\":\"ConnectorPlacement.EquallySpacedRectSide\",\"uuid\":\"9190d96c-22e3-4cc9-a507-8f094dc67743\"},{\"content\":{\"side\":\"TOP\"},\"type\":\"ConnectorPlacement.EquallySpacedRectSide\",\"uuid\":\"08b46875-eac1-4edb-b2eb-5598dd517a75\"}]},\"type\":\"ConnectorPlacement.EquallySpacedConnector\",\"uuid\":\"c8d2d02b-cf5a-431f-8876-22d36c8a9b33\"}],\"packageUris\":[\"http://schema.mathworks.com/mf0/Connector/R2020b\"],\"version\":\"1.0\"}"
  mriDirectory : Subsystem
      settings: PortSchema="{\"entries\":[{\"content\":{\"headerSize\":26,\"margin\":15,\"minimumSpacing\":25,\"sides\":[{\"content\":{},\"type\":\"ConnectorPlacement.EquallySpacedRectSide\",\"uuid\":\"d99db108-8c8a-4010-81b2-f142fbf318f5\"},{\"content\":{\"connectorIds\":[\"Out1\"],\"side\":\"RIGHT\"},\"type\":\"ConnectorPlacement.EquallySpacedRectSide\",\"uuid\":\"9190d96c-22e3-4cc9-a507-8f094dc67743\"},{\"content\":{\"side\":\"TOP\"},\"type\":\"ConnectorPlacement.EquallySpacedRectSide\",\"uuid\":\"08b46875-eac1-4edb-b2eb-5598dd517a75\"}]},\"type\":\"ConnectorPlacement.EquallySpacedConnector\",\"uuid\":\"c8d2d02b-cf5a-431f-8876-22d36c8a9b33\"}],\"packageUris\":[\"http://schema.mathworks.com/mf0/Connector/R2020b\"],\"version\":\"1.0\"}"
  mri_convert : Subsystem
      settings: PortSchema="{\"entries\":[{\"content\":{\"headerSize\":26,\"margin\":15,\"minimumSpacing\":25,\"sides\":[{\"content\":{\"connectorIds\":[\"In1\"]},\"type\":\"ConnectorPlacement.EquallySpacedRectSide\",\"uuid\":\"d99db108-8c8a-4010-81b2-f142fbf318f5\"},{\"content\":{\"connectorIds\":[\"Out1\",\"Out2\"],\"side\":\"RIGHT\"},\"type\":\"ConnectorPlacement.EquallySpacedRectSide\",\"uuid\":\"9190d96c-22e3-4cc9-a507-8f094dc67743\"},{\"content\":{\"side\":\"TOP\"},\"type\":\"ConnectorPlacement.EquallySpacedRectSide\",\"uuid\":\"08b46875-eac1-4edb-b2eb-5598dd517a75\"}]},\"type\":\"ConnectorPlacement.EquallySpacedConnector\",\"uuid\":\"c8d2d02b-cf5a-431f-8876-22d36c8a9b33\"}],\"packageUris\":[\"http://schema.mathworks.com/mf0/Connector/R2020b\"],\"version\":\"1.0\"}"
  scriptsDirectory : Subsystem
      settings: PortSchema="{\"entries\":[{\"content\":{\"headerSize\":26,\"margin\":15,\"minimumSpacing\":25,\"sides\":[{\"content\":{},\"type\":\"ConnectorPlacement.EquallySpacedRectSide\",\"uuid\":\"d99db108-8c8a-4010-81b2-f142fbf318f5\"},{\"content\":{\"connectorIds\":[\"Out1\"],\"side\":\"RIGHT\"},\"type\":\"ConnectorPlacement.EquallySpacedRectSide\",\"uuid\":\"9190d96c-22e3-4cc9-a507-8f094dc67743\"},{\"content\":{\"side\":\"TOP\"},\"type\":\"ConnectorPlacement.EquallySpacedRectSide\",\"uuid\":\"08b46875-eac1-4edb-b2eb-5598dd517a75\"}]},\"type\":\"ConnectorPlacement.EquallySpacedConnector\",\"uuid\":\"c8d2d02b-cf5a-431f-8876-22d36c8a9b33\"}],\"packageUris\":[\"http://schema.mathworks.com/mf0/Connector/R2020b\"],\"version\":\"1.0\"}"
  statsDirectory : Subsystem
      settings: PortSchema="{\"entries\":[{\"content\":{\"headerSize\":26,\"margin\":15,\"minimumSpacing\":25,\"sides\":[{\"content\":{},\"type\":\"ConnectorPlacement.EquallySpacedRectSide\",\"uuid\":\"d99db108-8c8a-4010-81b2-f142fbf318f5\"},{\"content\":{\"connectorIds\":[\"Out1\"],\"side\":\"RIGHT\"},\"type\":\"ConnectorPlacement.EquallySpacedRectSide\",\"uuid\":\"9190d96c-22e3-4cc9-a507-8f094dc67743\"},{\"content\":{\"side\":\"TOP\"},\"type\":\"ConnectorPlacement.EquallySpacedRectSide\",\"uuid\":\"08b46875-eac1-4edb-b2eb-5598dd517a75\"}]},\"type\":\"ConnectorPlacement.EquallySpacedConnector\",\"uuid\":\"c8d2d02b-cf5a-431f-8876-22d36c8a9b33\"}],\"packageUris\":[\"http://schema.mathworks.com/mf0/Connector/R2020b\"],\"version\":\"1.0\"}"
  subjectDirectory : Subsystem
      settings: PortSchema="{\"entries\":[{\"content\":{\"headerSize\":26,\"margin\":15,\"minimumSpacing\":25,\"sides\":[{\"content\":{\"connectorIds\":[\"In1\",\"In2\",\"In3\",\"In4\",\"In5\",\"In6\",\"In7\"]},\"type\":\"ConnectorPlacement.EquallySpacedRectSide\",\"uuid\":\"d99db108-8c8a-4010-81b2-f142fbf318f5\"},{\"content\":{\"connectorIds\":[\"Out1\"],\"side\":\"RIGHT\"},\"type\":\"ConnectorPlacement.EquallySpacedRectSide\",\"uuid\":\"9190d96c-22e3-4cc9-a507-8f094dc67743\"},{\"content\":{\"side\":\"TOP\"},\"type\":\"ConnectorPlacement.EquallySpacedRectSide\",\"uuid\":\"08b46875-eac1-4edb-b2eb-5598dd517a75\"}]},\"type\":\"ConnectorPlacement.EquallySpacedConnector\",\"uuid\":\"c8d2d02b-cf5a-431f-8876-22d36c8a9b33\"}],\"packageUris\":[\"http://schema.mathworks.com/mf0/Connector/R2020b\"],\"version\":\"1.0\"}"
  surfDirectory : Subsystem
      settings: PortSchema="{\"entries\":[{\"content\":{\"headerSize\":26,\"margin\":15,\"minimumSpacing\":25,\"sides\":[{\"content\":{},\"type\":\"ConnectorPlacement.EquallySpacedRectSide\",\"uuid\":\"d99db108-8c8a-4010-81b2-f142fbf318f5\"},{\"content\":{\"connectorIds\":[\"Out1\"],\"side\":\"RIGHT\"},\"type\":\"ConnectorPlacement.EquallySpacedRectSide\",\"uuid\":\"9190d96c-22e3-4cc9-a507-8f094dc67743\"},{\"content\":{\"side\":\"TOP\"},\"type\":\"ConnectorPlacement.EquallySpacedRectSide\",\"uuid\":\"08b46875-eac1-4edb-b2eb-5598dd517a75\"}]},\"type\":\"ConnectorPlacement.EquallySpacedConnector\",\"uuid\":\"c8d2d02b-cf5a-431f-8876-22d36c8a9b33\"}],\"packageUris\":[\"http://schema.mathworks.com/mf0/Connector/R2020b\"],\"version\":\"1.0\"}"
  tmpDirectory : Subsystem
      settings: PortSchema="{\"entries\":[{\"content\":{\"headerSize\":26,\"margin\":15,\"minimumSpacing\":25,\"sides\":[{\"content\":{},\"type\":\"ConnectorPlacement.EquallySpacedRectSide\",\"uuid\":\"d99db108-8c8a-4010-81b2-f142fbf318f5\"},{\"content\":{\"connectorIds\":[\"Out1\"],\"side\":\"RIGHT\"},\"type\":\"ConnectorPlacement.EquallySpacedRectSide\",\"uuid\":\"9190d96c-22e3-4cc9-a507-8f094dc67743\"},{\"content\":{\"side\":\"TOP\"},\"type\":\"ConnectorPlacement.EquallySpacedRectSide\",\"uuid\":\"08b46875-eac1-4edb-b2eb-5598dd517a75\"}]},\"type\":\"ConnectorPlacement.EquallySpacedConnector\",\"uuid\":\"c8d2d02b-cf5a-431f-8876-22d36c8a9b33\"}],\"packageUris\":[\"http://schema.mathworks.com/mf0/Connector/R2020b\"],\"version\":\"1.0\"}"
  trashDirectory : Subsystem
      settings: PortSchema="{\"entries\":[{\"content\":{\"headerSize\":26,\"margin\":15,\"minimumSpacing\":25,\"sides\":[{\"content\":{},\"type\":\"ConnectorPlacement.EquallySpacedRectSide\",\"uuid\":\"d99db108-8c8a-4010-81b2-f142fbf318f5\"},{\"content\":{\"connectorIds\":[\"Out1\"],\"side\":\"RIGHT\"},\"type\":\"ConnectorPlacement.EquallySpacedRectSide\",\"uuid\":\"9190d96c-22e3-4cc9-a507-8f094dc67743\"},{\"content\":{\"side\":\"TOP\"},\"type\":\"ConnectorPlacement.EquallySpacedRectSide\",\"uuid\":\"08b46875-eac1-4edb-b2eb-5598dd517a75\"}]},\"type\":\"ConnectorPlacement.EquallySpacedConnector\",\"uuid\":\"c8d2d02b-cf5a-431f-8876-22d36c8a9b33\"}],\"packageUris\":[\"http://schema.mathworks.com/mf0/Connector/R2020b\"],\"version\":\"1.0\"}"
  Bus Element Out1 : Outport  PortName=subject
  wires:
  Data1/1 -> mri_convert/1(Data)
  labelDirectory/1(label) -> subjectDirectory/7(label)
  scriptsDirectory/1(scripts) -> subjectDirectory/3(scripts)
  mriDirectory/1(mri) -> subjectDirectory/2(mri)
  trashDirectory/1(trash) -> subjectDirectory/6(trash)
  statsDirectory/1(stats) -> subjectDirectory/5(stats)
  surfDirectory/1(surf) -> subjectDirectory/4(surf)
  tmpDirectory/1(tmp) -> subjectDirectory/1(tmp)
  mri_convert/1(orig/002_mgz) -> autorecon1/2(orig/002_mgz)
  mri_convert/2(orig/001_mgz) -> autorecon1/1(orig/001_mgz)
  subjectDirectory/1(subject) -> Bus Element Out1/1

== system stormAD_Architecture_v1/Canada Compute Server/Remote Data Server/ sourceData ==
  Bus Element Out1 : Outport  AllowServiceAccess=on  PortName=remote

== system stormAD_Architecture_v1/Canada Compute Server/Remote Data Server/Home ==
  Bus Element Out1 : Outport  AllowServiceAccess=on  PortName=sourceCode

== system stormAD_Architecture_v1/Canada Compute Server/Remote Data Server/derivativesData ==

== system stormAD_Architecture_v1/Data Management/DataIngestor/Component ==
  Bus Element In2 : Inport  PortName=InBus
  Bus Element In1 : Inport  Port=2  PortName=multimodal
  Bus Element Out1 : Outport  PortName=OutBus

== system stormAD_Architecture_v1/Data Management/DataIngestor/getDerivatives ==
  Bus Element In1 : Inport  AllowServiceAccess=on  PortName=Derivatives Data
  Bus Element Out1 : Outport  PortName=multimodal

== system stormAD_Architecture_v1/Data Management/DataIngestor/getRawData ==
  Bus Element In1 : Inport  AllowServiceAccess=on  PortName=remote.raw
  Bus Element Out1 : Outport  PortName=multimodal

== system stormAD_Architecture_v1/Data Management/DataIngestor/readDataset ==
  Bus Element In1 : Inport  AllowServiceAccess=on  PortName=remote.raw
  Bus Element In2 : Inport  Port=2  AllowServiceAccess=on  PortName=remote.derivatives
  Bus Element Out1 : Outport  PortName=DatasetMap

== system stormAD_Architecture_v1/Data Management/Dataset ORM/DerivativesORM ==

== system stormAD_Architecture_v1/Data Management/Dataset ORM/RepoReader ==
  Bus Element In1 : Inport  PortName=UI-RepoFilePath
  cleanRepo : Subsystem
      settings: PortSchema="{\"entries\":[{\"content\":{\"headerSize\":26,\"margin\":15,\"minimumSpacing\":25,\"sides\":[{\"content\":{\"connectorIds\":[\"In1\"]},\"type\":\"ConnectorPlacement.EquallySpacedRectSide\",\"uuid\":\"a3539b9a-22db-4da3-b271-35b287ced3a1\"},{\"content\":{\"connectorIds\":[\"Out1\"],\"side\":\"RIGHT\"},\"type\":\"ConnectorPlacement.EquallySpacedRectSide\",\"uuid\":\"72d9f298-5062-46d4-b3c5-f2fa85d7a7a6\"},{\"content\":{\"side\":\"TOP\"},\"type\":\"ConnectorPlacement.EquallySpacedRectSide\",\"uuid\":\"050469fd-3881-4b53-a813-94df038aa659\"}]},\"type\":\"ConnectorPlacement.EquallySpacedConnector\",\"uuid\":\"6db04dad-62f3-4987-a6a9-d236db4fe2a3\"}],\"packageUris\":[\"http://schema.mathworks.com/mf0/Connector/R2020b\"],\"version\":\"1.0\"}"
  listDirectories : Subsystem
      settings: PortSchema="{\"entries\":[{\"content\":{\"headerSize\":26,\"margin\":15,\"minimumSpacing\":25,\"sides\":[{\"content\":{\"connectorIds\":[\"In1\"]},\"type\":\"ConnectorPlacement.EquallySpacedRectSide\",\"uuid\":\"a3539b9a-22db-4da3-b271-35b287ced3a1\"},{\"content\":{\"connectorIds\":[\"Out1\"],\"side\":\"RIGHT\"},\"type\":\"ConnectorPlacement.EquallySpacedRectSide\",\"uuid\":\"72d9f298-5062-46d4-b3c5-f2fa85d7a7a6\"},{\"content\":{\"side\":\"TOP\"},\"type\":\"ConnectorPlacement.EquallySpacedRectSide\",\"uuid\":\"050469fd-3881-4b53-a813-94df038aa659\"}]},\"type\":\"ConnectorPlacement.EquallySpacedConnector\",\"uuid\":\"6db04dad-62f3-4987-a6a9-d236db4fe2a3\"}],\"packageUris\":[\"http://schema.mathworks.com/mf0/Connector/R2020b\"],\"version\":\"1.0\"}"
  map : Subsystem
      settings: PortSchema="{\"entries\":[{\"content\":{\"headerSize\":26,\"margin\":15,\"minimumSpacing\":25,\"sides\":[{\"content\":{\"connectorIds\":[\"In1\"]},\"type\":\"ConnectorPlacement.EquallySpacedRectSide\",\"uuid\":\"a3539b9a-22db-4da3-b271-35b287ced3a1\"},{\"content\":{\"connectorIds\":[\"Out1\",\"Out2\"],\"side\":\"RIGHT\"},\"type\":\"ConnectorPlacement.EquallySpacedRectSide\",\"uuid\":\"72d9f298-5062-46d4-b3c5-f2fa85d7a7a6\"},{\"content\":{\"side\":\"TOP\"},\"type\":\"ConnectorPlacement.EquallySpacedRectSide\",\"uuid\":\"050469fd-3881-4b53-a813-94df038aa659\"}]},\"type\":\"ConnectorPlacement.EquallySpacedConnector\",\"uuid\":\"6db04dad-62f3-4987-a6a9-d236db4fe2a3\"}],\"packageUris\":[\"http://schema.mathworks.com/mf0/Connector/R2020b\"],\"version\":\"1.0\"}"
  Bus Element Out1 : Outport  PortName=RepoMap
  Bus Element Out2 : Outport  Port=2  PortName=syncrhonize_DB
  wires:
  Bus Element In1/1 -> listDirectories/1(UI-RepoFilePath)
  listDirectories/1(OutBus) -> cleanRepo/1(InBus)
  cleanRepo/1(OutBus) -> map/1(InBus)
  map/2(syncrhonize_DB) -> Bus Element Out2/1
  map/1(RepoMap) -> Bus Element Out1/1

== system stormAD_Architecture_v1/StormAD Core/MEG/featureExtractionModule ==

== system stormAD_Architecture_v1/StormAD Core/PET/PVC ==
  Bus Element In2 : Inport  PortName=maskUI
  Bus Element In1 : Inport  Port=2  PortName=InBus

== system stormAD_Architecture_v1/StormAD Core/PET/SUVR ==
  Bus Element In2 : Inport  PortName=regRegionUptake
  Bus Element In1 : Inport  Port=2  PortName=smoothedPET
  Bus Element Out1 : Outport  PortName=suvrVol
  Bus Element Out2 : Outport  Port=2  PortName=suvrVol2Proj

== system stormAD_Architecture_v1/StormAD Core/PET/T1finder ==
  Bus Element In1 : Inport  PortName=anat4pet
  Bus Element Out1 : Outport  PortName=T1

== system stormAD_Architecture_v1/StormAD Core/PET/align2anat ==
  Bus Element In1 : Inport  PortName=T1
  Bus Element In3 : Inport  Port=2  PortName=petFrames
  Bus Element Out1 : Outport  PortName=alignedFrames

== system stormAD_Architecture_v1/StormAD Core/PET/averagePET ==
  Bus Element In1 : Inport  PortName=alignedFrames
  Bus Element Out1 : Outport  PortName=averagedPET

== system stormAD_Architecture_v1/StormAD Core/PET/regionStat ==
  Bus Element In1 : Inport  PortName=refRegion
  Bus Element In3 : Inport  Port=2  PortName=maskUI
  Bus Element In4 : Inport  Port=3  PortName=smoothedPET2
  maskSelector : Subsystem
      settings: PortSchema="{\"entries\":[{\"content\":{\"headerSize\":26,\"margin\":15,\"minimumSpacing\":25,\"sides\":[{\"content\":{\"connectorIds\":[\"In1\",\"In2\"]},\"type\":\"ConnectorPlacement.EquallySpacedRectSide\",\"uuid\":\"a3539b9a-22db-4da3-b271-35b287ced3a1\"},{\"content\":{\"connectorIds\":[\"Out1\"],\"side\":\"RIGHT\"},\"type\":\"ConnectorPlacement.EquallySpacedRectSide\",\"uuid\":\"72d9f298-5062-46d4-b3c5-f2fa85d7a7a6\"},{\"content\":{\"side\":\"TOP\"},\"type\":\"ConnectorPlacement.EquallySpacedRectSide\",\"uuid\":\"050469fd-3881-4b53-a813-94df038aa659\"}]},\"type\":\"ConnectorPlacement.EquallySpacedConnector\",\"uuid\":\"6db04dad-62f3-4987-a6a9-d236db4fe2a3\"}],\"packageUris\":[\"http://schema.mathworks.com/mf0/Connector/R2020b\"],\"version\":\"1.0\"}"
  smoothedPET : Subsystem
      settings: PortSchema="{\"entries\":[{\"content\":{\"headerSize\":26,\"margin\":15,\"minimumSpacing\":25,\"sides\":[{\"content\":{\"connectorIds\":[\"In1\"]},\"type\":\"ConnectorPlacement.EquallySpacedRectSide\",\"uuid\":\"a3539b9a-22db-4da3-b271-35b287ced3a1\"},{\"content\":{\"side\":\"RIGHT\"},\"type\":\"ConnectorPlacement.EquallySpacedRectSide\",\"uuid\":\"72d9f298-5062-46d4-b3c5-f2fa85d7a7a6\"},{\"content\":{\"side\":\"TOP\"},\"type\":\"ConnectorPlacement.EquallySpacedRectSide\",\"uuid\":\"050469fd-3881-4b53-a813-94df038aa659\"}]},\"type\":\"ConnectorPlacement.EquallySpacedConnector\",\"uuid\":\"6db04dad-62f3-4987-a6a9-d236db4fe2a3\"}],\"packageUris\":[\"http://schema.mathworks.com/mf0/Connector/R2020b\"],\"version\":\"1.0\"}"
  Bus Element Out1 : Outport  PortName=regRegionUptake
  wires:
  Bus Element In3/1 -> maskSelector/1(maskUI)
  Bus Element In4/1 -> maskSelector/2(anat4pet)
  maskSelector/1(mask) -> smoothedPET/1(mask)

== system stormAD_Architecture_v1/StormAD Core/PET/smooth ==
  Bus Element In2 : Inport  PortName=smoothFactor
  Bus Element In1 : Inport  Port=2  PortName=averagedPET
  Bus Element Out2 : Outport  PortName=smoothedPET2
  Bus Element Out1 : Outport  Port=2  PortName=smoothedPET

== system stormAD_Architecture_v1/StormAD Core/PET/splitPET ==
  Bus Element In1 : Inport  PortName=pet
  Bus Element Out1 : Outport  PortName=petFrames

== system stormAD_Architecture_v1/StormAD Core/PET/surfFinder ==
  Bus Element In1 : Inport  PortName=anat4pet
  Bus Element Out1 : Outport  PortName=pial

== system stormAD_Architecture_v1/StormAD Core/PET/surfaceProjector ==
  Bus Element In3 : Inport  PortName=suvrVol2Proj
  Bus Element In2 : Inport  Port=2  PortName=surfParams
  Bus Element In1 : Inport  Port=3  PortName=pial
  Bus Element Out1 : Outport  PortName=suvrSurf

== system stormAD_Architecture_v1/StormAD Remote/Local WSL Store/bash Scripts ==

== system stormAD_Architecture_v1/StormAD Remote/Local WSL Store/slurm Jobs ==

== system stormAD_Architecture_v1/StormAD Remote/Local WSL Store/sshConnect ==
